simulink model "closedloopcontrol_PID"  (R2020a)
settings: Solver=VariableStepAuto  StartTime=0.0  StopTime=60  MaxStep=0.0001  RelTol=1e-3
model workspace (MAT data in the model file):
  C = 128
libraries: powerlib x4, ECEN315_Library x2, ECEN315_Library_motor_new x1
settings Model: Creator=burmesdani  LastModifiedBy=Daniel
settings DataIOCC: ReturnWorkspaceOutputs=off
settings DebuggingCC: ArithmeticOperatorsInVariantConditions=warning
settings SFSimCC: SimUseLocalCustomCode=off  CustomCodeUndefinedFunction=UseInterfaceOnly
settings RTWCC: RTWUseLocalCustomCode=off

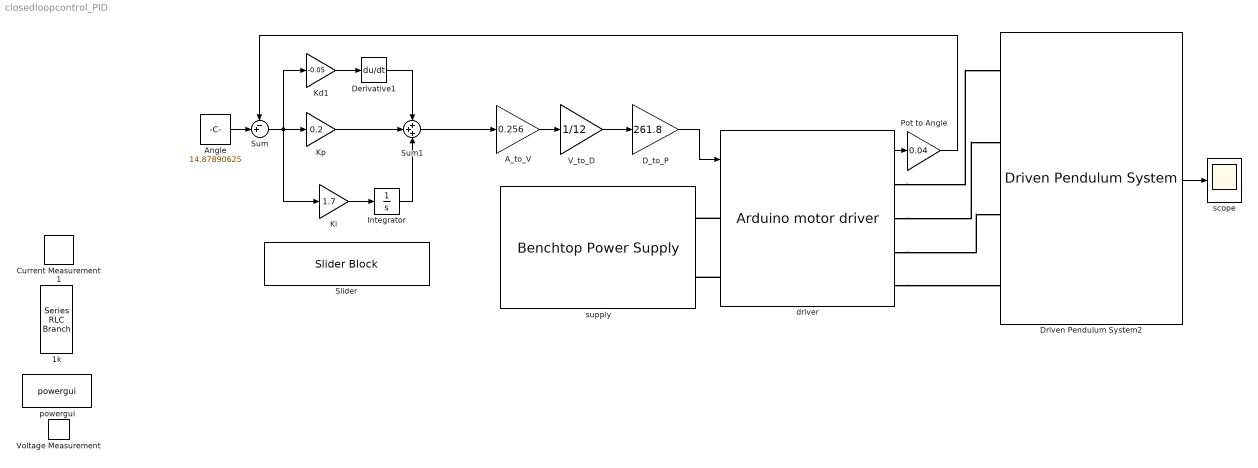
== system closedloopcontrol_PID ==
  1k : powerlib/Elements/Series RLC Branch  LConnTagsString=__new0  RConnTagsString=__new0  BranchType=R  Resistance=1000  Inductance=1e-3  SetiL0=off  InitialCurrent=0  Capacitance=1e-6  Setx0=off  InitialVoltage=0  Measurements=None
  A_to_V : Gain  Gain=0.256
  Angle : Constant  Value=14.87890625
  Current Measurement1 : powerlib/Measurements/Current Measurement  PhasorSimulation=off  OutputType=Complex  PSBequivalent=0
  D_to_P : Gain  Gain=261.8
  Derivative1 : Derivative
  Driven Pendulum System2 : ECEN315_Library/Driven Pendulum System  SystemSampleTime=-1  Latency=0  AutoFrameSizeCalculation=off
  Integrator : Integrator
  Kd1 : Gain  Gain=-0.05
  Ki : Gain  Gain=1.7
  Kp : Gain  Gain=0.2
  Pot to Angle : Gain  Gain=0.04
  Slider : SliderBlock  ScaleMax=45
  Sum : Sum  Inputs=-+|
  Sum1 : Sum  Inputs=+++
  V_to_D : Gain  Gain=1/12
  Voltage Measurement : powerlib/Measurements/Voltage Measurement  PhasorSimulation=off  OutputType=Complex  PSBequivalent=0
  driver : ECEN315_Library_motor_new/Arduino motor driver  E=on
  powergui : powerlib/powergui  Priority=1  SimulationMode=Continuous  SampleTime=50e-6  frequency=60  Iterations=50  frequencyindice=0  Pbase=100e6  ErrMax=1e-4  UnitsV=kV  UnitsW=MW  buscounter=0  FunctionMessages=off  echomessages=off  EnableUseOfTLC=off  CurrentSourceSwitches=off  DisableSnubberDevices=off  DisableRonSwitches=off  DisableVfSwitches=off  DisplayEquations=off  AutomaticDiscreteSolvers=off  SolverType=Tustin/Backward Euler (TBE)  Interpol=off  ExternalGateDelay=off  methode=off  Ts=100  x0status=blocks  SPID=on  SwTol=0  HookPort=off  NonlinearTolerance=1e-4  nMaxIteration=100  ContinueOnMaxIteration=off  RestoreLinks=warning  ResistiveCurrentMeasurement=off  Frange=[0:2:500]  Ylog=off  Xlog=on  ShowGrid=off  save=off  variable=ZData  structure=0  ZoomFFT=off  StartTime=0.0  cycles=1  DisplayStyle=1  fundamental=60  FreqAxis=off  MaxFrequency=1000  frequencyindicesteady=1  RmsSteady=1  display=off
  scope : Scope
  supply : ECEN315_Library/Benchtop Power Supply  V=12
  wires:
  Pot to Angle/1 -> Sum/1
  driver/1 -> Pot to Angle/1
  A_to_V/1 -> V_to_D/1
  V_to_D/1 -> D_to_P/1
  D_to_P/1 -> driver/1
  Driven Pendulum System2/1 -> scope/1
  Sum1/1 -> A_to_V/1
  Kp/1 -> Sum1/2
  Angle/1 -> Sum/2
  Derivative1/1 -> Sum1/1
  Kd1/1 -> Derivative1/1
  Integrator/1 -> Sum1/3
  Ki/1 -> Integrator/1
  Sum/1 -> Ki/1, Kd1/1, Kp/1
  connections:
  driver/LConn2 -- supply/RConn2
  driver/LConn1 -- supply/RConn1
  driver/RConn1 -- Driven Pendulum System2/LConn1
  driver/RConn4 -- Driven Pendulum System2/LConn4
  driver/RConn2 -- Driven Pendulum System2/LConn2
  driver/RConn3 -- Driven Pendulum System2/LConn3
